simulink library "dkc"  (R2021b)
settings: Solver=VariableStepAuto  StartTime=0.0  StopTime=10.0  RelTol=1e-3
undefined symbols (not defined in the file or in its folder): ENUM_ANTITHEFT_ALARM, ENUM_ANTITHEFT_ARM, ENUM_ANTITHEFT_DISARM, ENUM_ANTITHEFT_WAIT, ENUM_BTCONNSTA_CONNECTED, ENUM_BTConnSta_CONNECTED, ENUM_BTCONNSTA_DISCONNECTED, ENUM_DKCAuthSta_DECRYPTIONFAIL, ENUM_DKCAuthSta_NORMAL, ENUM_DKCAuthSta_TIMEERROR, ENUM_DKCPCMDHANDING_FORCELIFT, ENUM_DKCPCMDHANDING_LOCK, ENUM_DKCPCMDHANDING_LOCKTGATEFAIL, ENUM_DKCPCMDHANDING_OVER, ENUM_DKCPCMDHANDING_TGATEHANDLE, ENUM_DKCPCMDHANDING_UNLOCK, ENUM_DkeyShowIVI_DEFAULT, ENUM_DkeyShowIVI_INVALID, ENUM_DkeyShowIVI_NFCGREEN, ENUM_DkeyShowIVI_NFCRED, ENUM_GEARACTUALPOSN_N, ENUM_GEARACTUALPOSN_P, ENUM_KEYMISSSTA_DEFAULT, ENUM_KEYMISSSTA_KEYMISS, ENUM_KEYMODE_DAFAULT, ENUM_KEYMODE_INVALID, ENUM_KEYMODE_NFC, ENUM_KEYMODE_UIDBLE, ENUM_KEYMODE_UIDUWB, ENUM_KEYTYPE_NFC, ENUM_KEYTYPE_NOREQ, ENUM_KEYTYPE_UID, ENUM_PCMDTOBCM_DEFAULT, ENUM_PCMDTOBCM_FORCELIFT, ENUM_PCMDTOBCM_LOCK, ENUM_PCMDTOBCM_LOCKTGATEFAIL, ENUM_PCMDTOBCM_NFCCOMMAND, ENUM_PCMDTOBCM_REMOTETGATE, ENUM_PCMDTOBCM_TGATEHANDLE, ENUM_PCMDTOBCM_UNLOCK, ENUM_PCMDTOBCM_UWBLOCK, ENUM_PCMDTOBCM_UWBUNLOCK, ENUM_PDKEYPTGRAW_INTOZONE, ENUM_PDKEYPTGRAW_OUTZONE, ENUM_PDKEYPTGRAW_UNAVALIABLE, ENUM_PDKEYRAWLULOCK_INLOCK, ENUM_PDKEYRAWLULOCK_INUNLOCK, ENUM_PDKEYRAWLULOCK_UNAVALIABLE, ENUM_PDKEYRAWPS_INPS, ENUM_PDKEYRAWPS_OUTPS, ENUM_PDKEYRAWPS_UNAVALIABLE, ENUM_PDKEYSPTGRAW_INTOZONE, ENUM_PDKEYSPTGRAW_OUTZONE, ENUM_PDKEYSPTGRAW_UNAVALIABLE, ENUM_PDKEYWELCOMERAW_INTOZONE, ENUM_PDKEYWELCOMERAW_UNAVALIABLE, ENUM_POWERSTA_OFF, ENUM_POWERSTA_OFFA, ENUM_POWERSTA_OFFC, ENUM_POWERSTA_ON ... (+79)
libraries: simulink x99, hcu_lib x6
(part 1 of 4)
settings Model: Creator=Shawn  LastModifiedBy=FVT23010
settings SolverCC: AlgebraicLoopSolver=TrustRegion

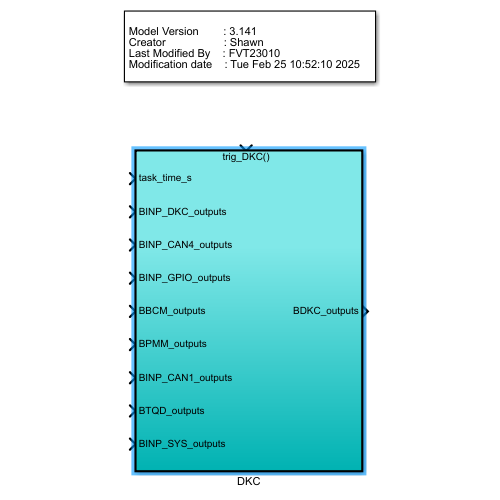
[thumbnail: Simulink's stored preview of the top-level diagram]
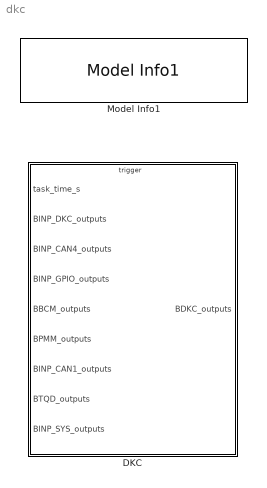
== system dkc ==
  DKC : Subsystem  TreatAsAtomicUnit=on
      settings: RTWSystemCode=Nonreusable function  RTWFcnNameOpts=Use subsystem name  RTWFileNameOpts=Use subsystem name
  Model Info1 : hcu_lib/Model Info1  BlockCM=None  Frame=on  DisplayStringWithTags=|  HorizontalTextAlignment=Left  LeftAlignmentValue=0.02  SourceBlockDiagram=hcu_lib  TagMaxNumber=20
      | Model Version        : %<ModelVersion>
      | Creator                   : %<Creator>
      | Last Modified By    : %<LastModifiedBy>
      | Modification date    : %<LastModificationDate>

== system dkc/DKC ==
  task_time_s : Inport
  BINP_DKC_outputs : Inport  Port=2  OutDataTypeStr=Bus: BINP_DKC_outputs
  BINP_CAN4_outputs : Inport  Port=3  OutDataTypeStr=Bus: BINP_CAN4_outputs
  BINP_GPIO_outputs : Inport  Port=4  OutDataTypeStr=Bus: BINP_GPIO_outputs
  BBCM_outputs : Inport  Port=5  OutDataTypeStr=Bus: BBCM_outputs
  BPMM_outputs : Inport  Port=6  OutDataTypeStr=Bus: BPMM_outputs
  BINP_CAN1_outputs : Inport  Port=7  OutDataTypeStr=Bus: BINP_CAN1_outputs
  BTQD_outputs : Inport  Port=8  OutDataTypeStr=Bus: BTQD_outputs
  BINP_SYS_outputs : Inport  Port=9  OutDataTypeStr=Bus: BINP_SYS_outputs
  trig_DKC : TriggerPort  TriggerType=function-call  VariantControl=(inherit)
  Subsystem : Subsystem
  BDKC_outputs : Outport  OutDataTypeStr=Bus: BDKC_outputs
  wires:
  BINP_SYS_outputs/1 -> Subsystem/9(BINP_SYS_outputs)
  BTQD_outputs/1 -> Subsystem/8(BTQD_outputs)
  BINP_CAN1_outputs/1 -> Subsystem/7(BINP_CAN1_outputs)
  BPMM_outputs/1 -> Subsystem/6(BPMM_outputs)
  BBCM_outputs/1 -> Subsystem/5(BBCM_outputs)
  BINP_GPIO_outputs/1 -> Subsystem/4(BINP_GPIO_outputs)
  BINP_CAN4_outputs/1 -> Subsystem/3(BINP_CAN4_outputs)
  Subsystem/1(BDKC_outputs) -> BDKC_outputs/1
  BINP_DKC_outputs/1 -> Subsystem/2(BINP_DKC_outputs)
  task_time_s/1 -> Subsystem/1(task_time_s)  "task_time_s"

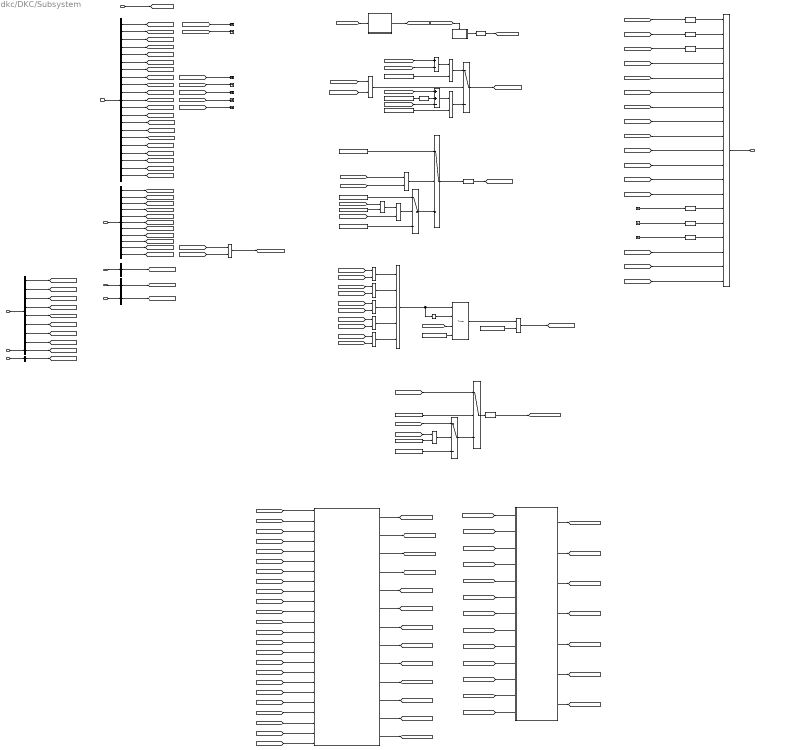
== system dkc/DKC/Subsystem ==
  note: DKC Authentication State
  note: Check DKCTimeSN
  note: DKC Time Serial Number
  note: FDC_DKC_KeyMiss_Sta
      | VDKC_KeyMissSta_flg
      |
      | FDC_DKC_KeyMode_Sta
      | VDKC_KeyModeSta_enum
      |
      | FDC_DKC_DkeyShowIVI_Sta
      | VDKC_DkeyShowIVISta_enum
      |
      | FDC_DKC_DKeyAreaPS_Sta
      | VDKC_KeyAreaPS_enum
      |
      | FDC_DKC_DKeyAreaPE_Sta
      | VDKC_KeyAreaLockUnlock_enum
      |
      | FDC_DKC_CommandToBCM_Cmd
      | VDKC_PCommandToBCM_enum
      |
      | FDC_DKC_DKeyWelcome_Sta
      | VDKC_DKeyWelcomeSta_enum
      |
      | FDC_DKC_ DKeyArea_PTG_Sta
      | VDKC_KeyAreaPTG_enum
      |
      | FDC_DKC_ DKeyArea_SPTG_Sta
      | VDKC_KeyAreaSPTGSta_enum
      |
      | FDC_DKC_ UIDLowPower_Sta
      | VDKC_UIDLowPowerSta_enum
      |
      | FDC_DKC_DkeyAreaRAPS_Sta
      | VDKC_DkeyAreaRAPSSta_enum
      |
      | FDC_DKC_ParkingMode_Cmd
      | VDKC_ParkingModeCmd_enum
      |
      | FDC_DKC_KeyNum_Sta
      | VDKC_KeyNumSta_enum
      |
      | FDC_DKC_KeyType_Sta
      | VDKC_KeyTypeSta_enum
  note: Compare plaintext and ciphertext
  task_time_s : Inport
  BINP_DKC_outputs : Inport  Port=2  OutDataTypeStr=Bus: BINP_DKC_outputs
  BINP_CAN4_outputs : Inport  Port=3  OutDataTypeStr=Bus: BINP_CAN4_outputs
  BINP_GPIO_outputs : Inport  Port=4
  BBCM_outputs : Inport  Port=5
  BPMM_outputs : Inport  Port=6
  BINP_CAN1_outputs : Inport  Port=7  OutDataTypeStr=Bus: BINP_CAN1_outputs
  BTQD_outputs : Inport  Port=8  OutDataTypeStr=Bus: BTQD_outputs
  BINP_SYS_outputs : Inport  Port=9  OutDataTypeStr=Bus: BINP_SYS_outputs
  Add : Sum  Inputs=+-
  Add3 : Sum  Inputs=++-
  Bus Creator : BusCreator  Inputs=19  OutDataTypeStr=Bus: BDKC_outputs  NonVirtualBus=on
  Bus Selector : BusSelector  OutputSignals=VINP_PCommandToBCM_enum,VINP_PCommandToPTG_enum,VINP_PDKeyAreaLockUnlock_enum,VINP_PDKeyAreaPS_enum,VINP_PDKeyAreaPTG_enum,VINP_BPPTGInsideSW2Sta_enum,VINP_BPPTGInsideSW1Sta_enum,VINP_CANMsgValidDKC1_flg,VINP_PDKeyWelcome_enum,VINP_CANMsgValidZONEDR1_flg,VINP_CANMsgValidZONEFR1_flg
  Bus Selector1 : BusSelector  OutputSignals=VINP_DKCDecReVehData_enum,VINP_DKCDecRemotePW_enum,VINP_DKCDecPCommandToBCM_enum,VINP_DKCDecPCommandToPTG_enum,VINP_DKCDecPDKeyAreaLockUnlock_enum,VINP_DKCDecPDKeyAreaPS_enum,VINP_DKCDecPDKeyAreaPTG_enum,VINP_DKCDecPDKeyWelcome_enum,VINP_DKCDecPDkeyShowIVI_enum,VINP_DKCDecPKeyMiss_flg,VINP_DKCDecPKeyMode_enum,VINP_DKCDecPUIDLowPower_flg,VINP_TimeSNDKCFbk_cnt,VINP_DKCDecryptionFail_flg,VINP_NFCDoorSta_flg,VINP_NFCLidASta_flg,VINP_KeyFobAreaU16_enum,VINP_UIDButtonCmd_enum,VINP_BTConnectSta_enum,VINP_UIDBatVoltx1000_V,VINP_DKCBTRSSI_dB
  Bus Selector2 : BusSelector  OutputSignals=VINP_DrDoorSW_flg,VINP_PsDoorSW_flg,VINP_RRDoorSW_flg,VINP_RLDoorSW_flg,VINP_TailgateSW_flg,VINP_TrunkHanSW_flg,VINP_BrakeSWGPIO_flg,VINP_SeatSW_flg
  Bus Selector3 : BusSelector  OutputSignals=VBCM_AntitheftSta_enum
  Bus Selector4 : BusSelector  OutputSignals=VPMM_PowerSta_enum
  Bus Selector5 : BusSelector  OutputSignals=VINP_VehSpeed_kph
  Bus Selector6 : BusSelector  OutputSignals=VTQD_GearActualPosn_enum
  Bus Selector7 : BusSelector  OutputSignals=VINP_FlashJugKeepUnLZone_flg
  Constant : Constant  Value=ENUM_DKCAuthSta_TIMEERROR
  Constant1 : Constant  Value=KDKC_DKCDecryptionErrorAllow_s
  Constant10 : Constant  Value=ENUM_DKCAuthSta_NORMAL
  Constant11 : Constant  Value=ENUM_PDKEYRAWLULOCK_UNAVALIABLE
  Constant2 : Constant  Value=0xFFFFFFFF
  Constant3 : Constant  Value=KDKC_TimeSNAllowDiff_cnt
  Constant4 : Constant  Value=KDKC_TimeSNAllowDiff_cnt
  Constant5 : Constant  Value=ENUM_DKCAuthSta_NORMAL
  Constant6 : Constant  Value=KDKC_InitialTimeErrorAllow_cnt
  Constant7 : Constant  Value=ENUM_DKCAuthSta_DECRYPTIONFAIL
  Constant8 : Constant  Value=KDKC_DKCDecryptionErrorAllow_s
  Constant9 : Constant  Value=KDKC_KeyModeSw_flg
  DKC_Handler : Subsystem
  DKC_Scheduler : Stateflow chart  TreatAsAtomicUnit=on
  Data Type Conversion{,3,5..6,17..18,23} (7 alike) : DataTypeConversion
  Data Type Conversion1 : DataTypeConversion  OutDataTypeStr=uint32
  Data Type Conversion4 : DataTypeConversion  OutDataTypeStr=uint8
  Data Type Conversion7 : DataTypeConversion  OutDataTypeStr=uint32
  Equal{,2,6..8} (5 alike) : RelationalOperator  Operator=~=  OutDataTypeStr=boolean  RndMeth=Simplest
  Equal{1,3..5} (4 alike) : RelationalOperator  Operator=<=  OutDataTypeStr=boolean  RndMeth=Simplest
  Equal10 : RelationalOperator  Operator===  OutDataTypeStr=boolean  RndMeth=Simplest
  Equal9 : RelationalOperator  OutDataTypeStr=boolean  RndMeth=Simplest
  Ground1 : Ground
  Ground2 : Ground
  Ground3 : Ground
  Logical Operator : Logic  Operator=OR  Inputs=5  AllPortsSameDT=off  OutDataTypeStr=boolean
  Logical Operator1 : Logic  Operator=OR  AllPortsSameDT=off  OutDataTypeStr=boolean
  Logical Operator2 : Logic  AllPortsSameDT=off  OutDataTypeStr=boolean
  Logical Operator3 : Logic  Operator=OR  AllPortsSameDT=off  OutDataTypeStr=boolean
  NOT : Logic  Operator=NOT  AllPortsSameDT=off  OutDataTypeStr=boolean
  Subsystem : Subsystem
  Switch{,1..4} (5 alike) : Switch  Criteria=u2 ~= 0
  Terminator{,1..6} (7 alike) : Terminator
  Timer : hcu_lib/Basic_Blocks/Timer
  Triggered Subsystem : Subsystem  TreatAsAtomicUnit=on
  BDKC_outputs : Outport
  wires:
  BINP_SYS_outputs/1 -> Bus Selector7/1
  [VINP_FlashJugKeepUnLZone_flg] -> DKC_Handler/24(VINP_FlashJugKeepUnLZone_flg)
  Bus Selector7/1 -> [VINP_FlashJugKeepUnLZone_flg]  "<VINP_FlashJugKeepUnLZone_flg>"
  DKC_Handler/13(VDKC_JudgeKeepUnlockZone_flg) -> [VDKC_JudgeKeepUnlockZone_flg]
  [VINP_DKCBTRSSI_dB] -> DKC_Handler/23(VINP_DKCBTRSSI_dB)
  [VINP_UIDBatVoltx1000_V] -> DKC_Handler/22(VINP_UIDBatVoltx1000_V)
  [VINP_BTConnectSta_enum] -> DKC_Handler/21(VINP_BTConnectSta_enum)
  Bus Selector1/21 -> [VINP_DKCBTRSSI_dB]  "<VINP_DKCBTRSSI_dB>"
  Bus Selector1/20 -> [VINP_UIDBatVoltx1000_V]  "<VINP_UIDBatVoltx1000_V>"
  Bus Selector1/19 -> [VINP_BTConnectSta_enum]  "<VINP_BTConnectSta_enum>"
  Bus Selector2/7 -> [VINP_BrakeSWGPIO_flg]  "<VINP_BrakeSWGPIO_flg>"
  Bus Selector/9 -> [VINP_PDKeyWelcome_enum]  "<VINP_PDKeyWelcome_enum>"
  Bus Selector/8 -> [VINP_CANMsgValidDKC1_flg]  "<VINP_CANMsgValidDKC1_flg>"
  Ground3/1 -> Data Type Conversion18/1
  Ground2/1 -> Data Type Conversion6/1
  Ground1/1 -> Data Type Conversion3/1
  Bus Selector2/6 -> [VINP_TrunkHanSW_flg]  "<VINP_TrunkHanSW_flg>"
  Bus Selector/7 -> [VINP_BPPTGInsideSW1Sta_enum]  "<VINP_BPPTGInsideSW1Sta_enum>"
  Bus Selector/6 -> [VINP_BPPTGInsideSW2Sta_enum]  "<VINP_BPPTGInsideSW2Sta_enum>"
  Bus Selector6/1 -> [VTQD_GearActualPosn_enum]  "<VTQD_GearActualPosn_enum>"
  BTQD_outputs/1 -> Bus Selector6/1
  Bus Selector5/1 -> [VINP_VehSpeed_kph]  "<VINP_VehSpeed_kph>"
  BINP_CAN1_outputs/1 -> Bus Selector5/1
  Bus Selector1/18 -> [VINP_UIDButtonCmd_enum]  "<VINP_UIDButtonCmd_enum>"
  Bus Selector1/17 -> [VINP_KeyFobAreaU16_enum]  "<VINP_KeyFobAreaU16_enum>"
  Bus Selector1/16 -> [VINP_NFCLidASta_flg]  "<VINP_NFCLidASta_flg>"
  Bus Selector1/15 -> [VINP_NFCDoorSta_flg]  "<VINP_NFCDoorSta_flg>"
  Bus Selector3/1 -> [VBCM_AntitheftSta_enum]  "<VBCM_AntitheftSta_enum>"
  Bus Selector4/1 -> [VPMM_PowerSta_enum]  "<VPMM_PowerSta_enum>"
  Bus Selector2/5 -> [VINP_TailgateSW_flg]  "<VINP_TailgateSW_flg>"
  Bus Selector2/4 -> [VINP_RLDoorSW_flg]  "<VINP_RLDoorSW_flg>"
  Bus Selector2/2 -> [VINP_PsDoorSW_flg]  "<VINP_PsDoorSW_flg>"
  Bus Selector2/1 -> [VINP_DrDoorSW_flg]  "<VINP_DrDoorSW_flg>"
  Bus Selector2/3 -> [VINP_RRDoorSW_flg]  "<VINP_RRDoorSW_flg>"
  BPMM_outputs/1 -> Bus Selector4/1
  BBCM_outputs/1 -> Bus Selector3/1
  BINP_GPIO_outputs/1 -> Bus Selector2/1
  Bus Selector/5 -> [VINP_PDKeyAreaPTG_enum]  "<VINP_PDKeyAreaPTG_enum>"
  Bus Selector/4 -> [VINP_PDKeyAreaPS_enum]  "<VINP_PDKeyAreaPS_enum>"
  Bus Selector/3 -> [VINP_PDKeyAreaLockUnlock_enum]  "<VINP_PDKeyAreaLockUnlock_enum>"
  Bus Selector/2 -> [VINP_PCommandToPTG_enum]  "<VINP_PCommandToPTG_enum>"
  Bus Selector/1 -> [VINP_PCommandToBCM_enum]  "<VINP_PCommandToBCM_enum>"
  BINP_CAN4_outputs/1 -> Bus Selector/1
  Bus Selector1/14 -> [VINP_DKCDecryptionFail_flg]  "<VINP_DKCDecryptionFail_flg>"
  Switch1/1 -> Data Type Conversion4/1
  Constant6/1 -> Equal1/2
  [VDKC_DKCTimeSNCorrect_flg] -> Logical Operator1/2
  [VDKC_DKCTimeSN_cnt] -> Equal1/1
  Constant7/1 -> Switch1/1
  Data Type Conversion4/1 -> [VDKC_DKCAuthSta_enum]
  Switch/1 -> Switch1/3
  Equal1/1 -> Logical Operator1/1
  Logical Operator1/1 -> Switch/2
  Constant5/1 -> Switch/1
  Constant/1 -> Switch/3
  Constant3/1 -> Equal5/2
  [VINP_TimeSNDKCFbk_cnt] -> Add3/3
  Add3/1 -> Equal5/1
  Data Type Conversion1/1 -> Add3/2
  Constant2/1 -> Data Type Conversion1/1
  [VDKC_DKCTimeSN_cnt] -> Add3/1
  [VINP_TimeSNDKCFbk_cnt] -> Equal4/2
  [VDKC_DKCAuthSta_enum] -> Data Type Conversion5/1
  Data Type Conversion5/1 -> Bus Creator/2  "VDKC_DKCAuthSta_enum"
  [VINP_TimeSNDKCFbk_cnt] -> Data Type Conversion17/1
  [VDKC_DKCTimeSN_cnt] -> Data Type Conversion/1
  Data Type Conversion/1 -> Bus Creator/1  "VDKC_DKCTimeSN_cnt"
  Bus Creator/1 -> BDKC_outputs/1  "BDKC_outputs"
  Bus Selector1/13 -> [VINP_TimeSNDKCFbk_cnt]  "<VINP_TimeSNDKCFbk_cnt>"
  Bus Selector1/12 -> [VINP_DKCDecPUIDLowPower_flg]  "<VINP_DKCDecPUIDLowPower_flg>"
  Bus Selector1/11 -> [VINP_DKCDecPKeyMode_enum]  "<VINP_DKCDecPKeyMode_enum>"
  Bus Selector1/10 -> [VINP_DKCDecPKeyMiss_flg]  "<VINP_DKCDecPKeyMiss_flg>"
  Bus Selector1/9 -> [VINP_DKCDecPDkeyShowIVI_enum]  "<VINP_DKCDecPDkeyShowIVI_enum>"
  Bus Selector1/8 -> [VINP_DKCDecPDKeyWelcome_enum]  "<VINP_DKCDecPDKeyWelcome_enum>"
  Bus Selector1/7 -> [VINP_DKCDecPDKeyAreaPTG_enum]  "<VINP_DKCDecPDKeyAreaPTG_enum>"
  Bus Selector1/6 -> [VINP_DKCDecPDKeyAreaPS_enum]  "<VINP_DKCDecPDKeyAreaPS_enum>"
  Bus Selector1/5 -> [VINP_DKCDecPDKeyAreaLockUnlock_enum]  "<VINP_DKCDecPDKeyAreaLockUnlock_enum>"
  Bus Selector1/4 -> [VINP_DKCDecPCommandToPTG_enum]  "<VINP_DKCDecPCommandToPTG_enum>"
  Bus Selector1/3 -> [VINP_DKCDecPCommandToBCM_enum]  "<VINP_DKCDecPCommandToBCM_enum>"
  Bus Selector1/2 -> [VINP_DKCDecRemotePW_enum]  "<VINP_DKCDecRemotePW_enum>"
  Bus Selector1/1 -> [VINP_DKCDecReVehData_enum]  "<VINP_DKCDecReVehData_enum>"
  [VDKC_DKCTimeSN_cnt] -> Add/1
  Data Type Conversion7/1 -> [VDKC_DKCTimeSN_cnt]
  Triggered Subsystem/1(DKCTimeSN) -> Data Type Conversion7/1
  Switch2/1 -> [VDKC_DKCTimeSNCorrect_flg]  "VDKC_DKCTimeSNCorrect_flg"
  [task_time_s] -> DKC_Scheduler/1(task_time_s)
  Equal5/1 -> Switch2/3
  Equal3/1 -> Switch2/1
  Equal4/1 -> Switch2/2
  [VINP_TimeSNDKCFbk_cnt] -> Equal4/1
  Constant4/1 -> Equal3/2
  Add/1 -> Equal3/1
  [VINP_TimeSNDKCFbk_cnt] -> Add/2
  BINP_DKC_outputs/1 -> Bus Selector1/1
  [trig_DKCcounter_100ms] -> Triggered Subsystem/Trigger
  DKC_Scheduler/1(trig_DKCcounter_100ms()) -> [trig_DKCcounter_100ms]
  task_time_s/1 -> [task_time_s]
  Bus Selector/10 -> [VINP_CANMsgValidZONEDR1_flg]  "<VINP_CANMsgValidZONEDR1_flg>"
  Bus Selector/11 -> [VINP_CANMsgValidZONEFR1_flg]  "<VINP_CANMsgValidZONEFR1_flg>"
  [VINP_CANMsgValidZONEFR1_flg] -> Logical Operator2/2
  Logical Operator2/1 -> [VDKC_CANMsgValidZONEDRFR_flg]  "VDKC_CANMsgValidZONEDRFR_flg"
  [VINP_CANMsgValidZONEDR1_flg] -> Logical Operator2/1
  [VDKC_DKCDecryptionError_flg] -> Logical Operator3/2
  Logical Operator3/1 -> Switch1/2
  [VINP_DKCDecryptionFail_flg] -> Logical Operator3/1
  Logical Operator/1 -> Timer/1, NOT/1
  [VINP_DKCDecPCommandToBCM_enum] -> Equal/2
  [VINP_PCommandToBCM_enum] -> Equal/1
  Constant1/1 -> Equal9/2
  [VINP_DKCDecPDKeyAreaLockUnlock_enum] -> Equal6/2
  NOT/1 -> Timer/2
  Timer/1 -> Equal9/1
  Equal8/1 -> Logical Operator/5
  [VINP_DKCDecPDKeyAreaPTG_enum] -> Equal8/2
  Equal6/1 -> Logical Operator/3
  [task_time_s] -> Timer/3
  Equal2/1 -> Logical Operator/2
  Constant8/1 -> Timer/4
  [VINP_DKCDecPDKeyAreaPS_enum] -> Equal7/2
  Equal/1 -> Logical Operator/1
  Equal9/1 -> [VDKC_DKCDecryptionError_flg]  "VDKC_DKCDecryptionError_flg"
  [VINP_DKCDecPCommandToPTG_enum] -> Equal2/2
  [VINP_PCommandToPTG_enum] -> Equal2/1
  [VINP_PDKeyAreaPTG_enum] -> Equal8/1
  Equal7/1 -> Logical Operator/4
  [VINP_PDKeyAreaPS_enum] -> Equal7/1
  [VINP_PDKeyAreaLockUnlock_enum] -> Equal6/1
  Constant10/1 -> Equal10/2
  Constant9/1 -> Switch3/2
  Equal10/1 -> Switch4/2
  [VINP_DKCDecPDKeyAreaPS_enum] -> Switch4/1
  Switch4/1 -> Switch3/3
  Constant11/1 -> Switch4/3
  Data Type Conversion23/1 -> [VDKC_CAN4PDKeyAreaPS_enum]  "VDKC_CAN4PDKeyAreaPS_enum"
  [VDKC_DKCAuthSta_enum] -> Equal10/1
  [VINP_PDKeyAreaPS_enum] -> Switch3/1
  Switch3/1 -> Data Type Conversion23/1
  Data Type Conversion17/1 -> Bus Creator/3  "VDKC_TimeSNDKCFbk_cnt"
  Data Type Conversion3/1 -> Bus Creator/16  "VDKC_KeyNumSta_enum"
  Data Type Conversion6/1 -> Bus Creator/15  "VDKC_ParkingModeCmd_enum"
  Data Type Conversion18/1 -> Bus Creator/14  "VDKC_DkeyAreaRAPSSta_enum"
  [VDKC_KeyAreaSPTGSta_enum] -> Bus Creator/12
  [VDKC_KeyAreaPTG_enum] -> Bus Creator/11
  [VDKC_DKeyWelcomeSta_enum] -> Bus Creator/10
  [VDKC_PCommandToBCM_enum] -> Bus Creator/9
  [VDKC_KeyAreaLockUnlock_enum] -> Bus Creator/8
  [VDKC_KeyAreaPS_enum] -> Bus Creator/7
  [VDKC_DkeyShowIVISta_enum] -> Bus Creator/6
  DKC_Handler/7(VDKC_FDCKeyAllowSleep_flg) -> [VDKC_FDCKeyAllowSleep_flg]
  [VDKC_CANMsgValidZONEDRFR_flg] -> DKC_Handler/19(VDKC_CANMsgValidZONEDRFR_flg)
  DKC_Handler/5(VDKC_FDCKeyAreaSPTG_enum) -> [VDKC_FDCKeyAreaSPTG_enum]
  [VINP_BPPTGInsideSW2Sta_enum] -> DKC_Handler/17(VINP_BPPTGInsideSW2Sta_enum)
  [VINP_BPPTGInsideSW1Sta_enum] -> DKC_Handler/16(VINP_BPPTGInsideSW1Sta_enum)
  [VINP_TrunkHanSW_flg] -> DKC_Handler/15(VINP_TrunkHanSW_flg)
  [VTQD_GearActualPosn_enum] -> DKC_Handler/14(VTQD_GearActualPosn_enum)
  [VINP_VehSpeed_kph] -> DKC_Handler/13(VINP_VehSpeed_kph)
  DKC_Handler/4(VDKC_FDCKeyAreaPTG_enum) -> [VDKC_FDCKeyAreaPTG_enum]
  [VINP_UIDButtonCmd_enum] -> DKC_Handler/12(VINP_UIDButtonCmd_enum)
  [VINP_KeyFobAreaU16_enum] -> DKC_Handler/11(VINP_KeyFobAreaU16_enum)
  DKC_Handler/1(VDKC_FDCPCommandToBCM_enum) -> [VDKC_FDCPCommandToBCM_enum]
  DKC_Handler/2(VDKC_FDCKeyAreaLockUnlock_enum) -> [VDKC_FDCKeyAreaLockUnlock_enum]
  DKC_Handler/3(VDKC_FDCKeyAreaPS_enum) -> [VDKC_FDCKeyAreaPS_enum]
  [task_time_s] -> DKC_Handler/1(task_time_s)
  [VPMM_PowerSta_enum] -> DKC_Handler/10(VPMM_PowerSta_enum)
  [VBCM_AntitheftSta_enum] -> DKC_Handler/9(VBCM_AntitheftSta_enum)
  [VINP_TailgateSW_flg] -> DKC_Handler/8(VINP_TailgateSW_flg)
  [VINP_RLDoorSW_flg] -> DKC_Handler/7(VINP_RLDoorSW_flg)
  [VINP_RRDoorSW_flg] -> DKC_Handler/6(VINP_RRDoorSW_flg)
  [VINP_PsDoorSW_flg] -> DKC_Handler/5(VINP_PsDoorSW_flg)
  [VINP_DrDoorSW_flg] -> DKC_Handler/4(VINP_DrDoorSW_flg)
  [VINP_NFCDoorSta_flg] -> DKC_Handler/3(VINP_NFCDoorSta_flg)
  [VINP_NFCLidASta_flg] -> DKC_Handler/2(VINP_NFCLidASta_flg)
  DKC_Handler/6(VDKC_FDCKeyWelcomeSta_enum) -> [VDKC_FDCKeyWelcomeSta_enum]
  DKC_Handler/12(VDKC_DkeyShowIVISta_enum) -> [VDKC_DkeyShowIVISta_enum]
  [VINP_BrakeSWGPIO_flg] -> DKC_Handler/18(VINP_BrakeSWGPIO_flg)
  Subsystem/7(VDKC_FDCDKCAllowSleep_flg) -> [VDKC_FDCDKCAllowSleep_flg]
  [VDKC_FDCKeyAllowSleep_flg] -> Subsystem/13(VDKC_FDCKeyAllowSleep_flg)
  [VDKC_FDCKeyAreaSPTG_enum] -> Subsystem/11(VDKC_FDCKeyAreaSPTG_enum)
  Subsystem/5(VDKC_KeyAreaSPTGSta_enum) -> [VDKC_KeyAreaSPTGSta_enum]
  [VDKC_FDCPCommandToBCM_enum] -> Subsystem/7(VDKC_FDCPCommandToBCM_enum)
  [VINP_PDKeyAreaPTG_enum] -> Subsystem/5(VINP_PDKeyAreaPTG_enum)
  [VINP_CANMsgValidDKC1_flg] -> Subsystem/1(VINP_CANMsgValidDKC1_flg)
  Subsystem/1(VDKC_PCommandToBCM_enum) -> [VDKC_PCommandToBCM_enum]
  Subsystem/2(VDKC_KeyAreaLockUnlock_enum) -> [VDKC_KeyAreaLockUnlock_enum]
  Subsystem/3(VDKC_KeyAreaPS_enum) -> [VDKC_KeyAreaPS_enum]
  Subsystem/4(VDKC_KeyAreaPTG_enum) -> [VDKC_KeyAreaPTG_enum]
  [VDKC_FDCKeyAreaPTG_enum] -> Subsystem/10(VDKC_FDCKeyAreaPTG_enum)
  [VDKC_FDCKeyAreaLockUnlock_enum] -> Subsystem/8(VDKC_FDCKeyAreaLockUnlock_enum)
  [VDKC_FDCKeyAreaPS_enum] -> Subsystem/9(VDKC_FDCKeyAreaPS_enum)
  [VINP_PCommandToBCM_enum] -> Subsystem/2(VINP_PCommandToBCM_enum)
  [VINP_PDKeyAreaLockUnlock_enum] -> Subsystem/3(VINP_PDKeyAreaLockUnlock_enum)
  [VDKC_CAN4PDKeyAreaPS_enum] -> Subsystem/4(VINP_PDKeyAreaPS_enum)
  [VINP_PDKeyWelcome_enum] -> Subsystem/6(VINP_PDKeyWelcome_enum)
  Subsystem/6(VDKC_DKeyWelcomeSta_enum) -> [VDKC_DKeyWelcomeSta_enum]
  [VDKC_FDCKeyWelcomeSta_enum] -> Subsystem/12(VDKC_FDCKeyWelcomeSta_enum)
  [VDKC_FDCDKCAllowSleep_flg] -> Bus Creator/18
  [VINP_DKCDecReVehData_enum] -> Terminator/1
  [VINP_DKCDecRemotePW_enum] -> Terminator1/1
  [VINP_DKCDecPDKeyWelcome_enum] -> Terminator2/1
  [VINP_DKCDecPDkeyShowIVI_enum] -> Terminator3/1
  [VINP_DKCDecPKeyMiss_flg] -> Terminator4/1
  [VINP_DKCDecPKeyMode_enum] -> Terminator5/1
  [VINP_DKCDecPUIDLowPower_flg] -> Terminator6/1
  DKC_Handler/9(VDKC_UIDLowPowerSta_enum) -> [VDKC_UIDLowPowerSta_enum]
  DKC_Handler/8(VDKC_KeyMissSta_flg) -> [VDKC_KeyMissSta_flg]
  [VDKC_UIDLowPowerSta_enum] -> Bus Creator/13
  [VDKC_KeyMissSta_flg] -> Bus Creator/4
  [VDKC_KeyModeSta_enum] -> Bus Creator/5
  [VDKC_KeyTypeSta_enum] -> Bus Creator/17
  DKC_Handler/10(VDKC_KeyModeSta_enum) -> [VDKC_KeyModeSta_enum]
  DKC_Handler/11(VDKC_KeyTypeSta_enum) -> [VDKC_KeyTypeSta_enum]
  [VINP_SeatSW_flg] -> DKC_Handler/20(VINP_SeatSW_flg)
  Bus Selector2/8 -> [VINP_SeatSW_flg]  "<VINP_SeatSW_flg>"
  [VDKC_JudgeKeepUnlockZone_flg] -> Bus Creator/19
